simulink model "differentialDrive"  (R2022a)
settings: Solver=VariableStepAuto  StartTime=0.0  StopTime=10.0  RelTol=1e-3
settings Model: Creator=rodri  LastModifiedBy=rodri

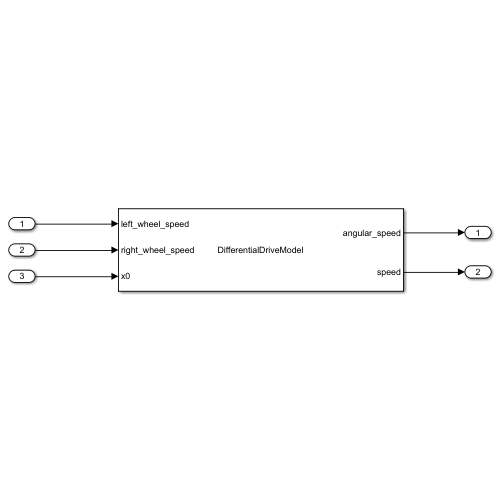
[thumbnail: Simulink's stored preview of the top-level diagram]
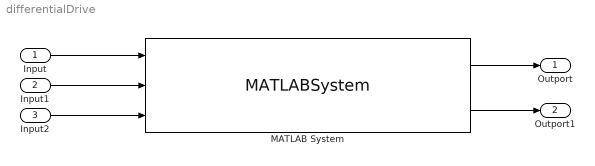
== system differentialDrive ==
  Input : Inport
  Input1 : Inport  Port=2
  Input2 : Inport  Port=3
  MATLAB System : MATLABSystem  System=DifferentialDriveModel  wheel_radius=1  wheel_base=1  x0=0  y0=0  theta0=0  SimulateUsing=Code generation
      mask Type: DifferentialDriveModel
      mask Display:
      | disp('DifferentialDriveModel');
      | port_label('input',1,'left_wheel_speed');
      | port_label('input',2,'right_wheel_speed');
      | port_label('input',3,'x0');
      | port_label('output',1,'angular_speed');
      | port_label('output',2,'speed');
  Outport : Outport
  Outport1 : Outport  Port=2
  wires:
  Input2/1 -> MATLAB System/3
  Input1/1 -> MATLAB System/2
  Input/1 -> MATLAB System/1
  MATLAB System/1 -> Outport/1
  MATLAB System/2 -> Outport1/1
